simulink subsystem "star_sensor"  (R2022b)
settings: Solver=VariableStepAuto  StartTime=0.0  StopTime=10.0  RelTol=1e-3
undefined symbols (not defined in the file or in its folder): catalogue, sat, sensors
libraries: simulink_extras x1
settings Model: Creator=brent  LastModifiedBy=brent

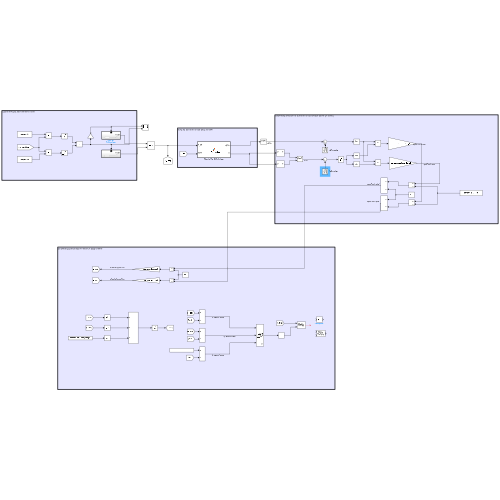
[thumbnail: Simulink's stored preview of the top-level diagram]
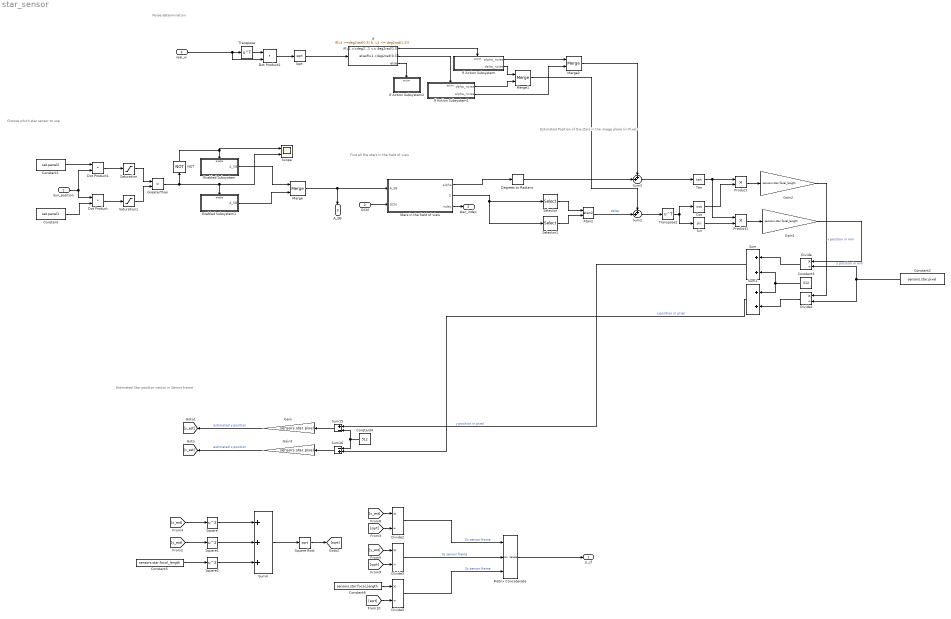
== system star_sensor ==
  note: Noise determination
  note: Estimated Star position vector in Sensor frame
  note: Estimated Position of the stars in the image plane (in Pixel)
  note: Find all the stars in the field of view
  note: Choose which star sensor to use
  Sun_position : Inport
  DCM : Inport  Port=2
  real_w : Inport  Port=3
  Atan2 : Trigonometry  Operator=atan2
  Constant : Constant  Value=sat.panel1
  Constant1 : Constant  Value=sat.panel2
  Constant2 : Constant  Value=sensors.star.pixel
  Constant3 : Constant  Value=512
  Constant4 : Constant  Value=512
  Constant5 : Constant  Value=sensors.star.focal_length
  Constant6 : Constant  Value=sensors.star.focal_length
  Cos : Trigonometry  Operator=cos
  Degrees to Radians : simulink_extras/Transformations/Degrees to Radians
  Divide{,1..3,5} (5 alike) : Product  Inputs=*/
  Dot Product : DotProduct  OutDataTypeStr=Inherit: Inherit via internal rule
  Dot Product1 : DotProduct  OutDataTypeStr=Inherit: Inherit via internal rule
  Dot Product2 : DotProduct  OutDataTypeStr=Inherit: Inherit via internal rule
  Enabled Subsystem : Subsystem  TreatAsAtomicUnit=on
  Enabled Subsystem1 : Subsystem  TreatAsAtomicUnit=on
  Gain : Gain  Gain=sensors.star.pixel
  Gain1 : Gain  Gain=sensors.star.focal_length
  Gain2 : Gain  Gain=sensors.star.focal_length
  Gain3 : Gain  Gain=sensors.star.pixel
  GreaterThan : RelationalOperator  Operator=>  OutDataTypeStr=boolean  RndMeth=Simplest  InputSameDT=off
  If : If  IfExpression="u1 >=deg2rad(0.3) &  u1 <= deg2rad(1.5)"  ElseIfExpressions=u1 <deg2rad(0.3)
  If Action Subsystem : Subsystem  TreatAsAtomicUnit=on
  If Action Subsystem1 : Subsystem  TreatAsAtomicUnit=on
  If Action Subsystem2 : Subsystem  TreatAsAtomicUnit=on
  Matrix Concatenate : Concatenate  NumInputs=3  Mode=Multidimensional array  ConcatenateDimension=2
  Merge : Merge
  Merge1 : Merge
  Merge2 : Merge
  NOT : Logic  Operator=NOT  IconShape=distinctive  AllPortsSameDT=off  OutDataTypeStr=boolean
  Product : Product
  Product1 : Product
  Saturation : Saturate  UpperLimit=1  LowerLimit=0
  Saturation1 : Saturate  UpperLimit=1  LowerLimit=0
  Scope : Scope  NumInputPorts=2
  Selector : Selector  NumberOfDimensions=2  InputPortWidth=3  IndexOptions=Index vector (dialog),Index vector (dialog)  Indices=2,[1:10]  OutputSizes=1,1
  Selector1 : Selector  NumberOfDimensions=2  InputPortWidth=3  IndexOptions=Index vector (dialog),Index vector (dialog)  Indices=1,[1:10]  OutputSizes=1,1
  Sin : Trigonometry
  Sqrt : Sqrt
  Square : Math  Operator=square
  Square Root : Sqrt
  Square1 : Math  Operator=square
  Square2 : Math  Operator=square
  Stars in the field of view : MATLAB Function  TreatAsAtomicUnit=on
  Sum : Sum
  Sum1 : Sum
  Sum15 : Sum  Inputs=+-
  Sum16 : Sum  Inputs=-+
  Sum2 : Sum  Inputs=++|
  Sum3 : Sum  Inputs=++|
  Sum4 : Sum  Inputs=+++
  Tan : Trigonometry  Operator=tan
  Transpose : Math  Operator=transpose
  Transpose2 : Math  Operator=transpose
  si_sf : Outport
  star_index : Outport  Port=2
  A_SB : Outport  Port=3
  wires:
  DCM/1 -> Stars in the field of view/2(DCM)
  Sun_position/1 -> Dot Product/1, Dot Product1/2
  Constant/1 -> Dot Product/2
  Dot Product/1 -> Saturation1/1
  Dot Product1/1 -> Saturation/1
  Constant1/1 -> Dot Product1/1
  Saturation/1 -> GreaterThan/1
  Saturation1/1 -> GreaterThan/2
  GreaterThan/1 -> NOT/1, Enabled Subsystem1/Enable, Scope/2
  NOT/1 -> Enabled Subsystem/Enable, Scope/1
  Enabled Subsystem/1(A_SB) -> Merge/1
  Enabled Subsystem1/1(A_SB) -> Merge/2
  Merge/1 -> Stars in the field of view/1(A_SB), A_SB/1
  Stars in the field of view/1(alpha) -> Degrees to Radians/1
  Tan/1 -> Product/1, Product1/1
  Cos/1 -> Product/2
  Sin/1 -> Product1/2
  Product1/1 -> Gain1/1
  Product/1 -> Gain2/1
  Gain2/1 -> Divide1/1  "x position in mm"
  Gain1/1 -> Divide/1  "y position in mm"
  Constant2/1 -> Divide1/2, Divide/2
  Constant3/1 -> Sum1/1, Sum/2
  Divide1/1 -> Sum1/2
  Divide/1 -> Sum/1
  Sum/1 -> Sum15/1  "y position in pixel"
  Sum1/1 -> Sum16/2  "x position in pixel"
  Stars in the field of view/2(S) -> Selector/1, Selector1/1
  Constant4/1 -> Sum16/1, Sum15/2
  Sum15/1 -> Gain/1
  Sum16/1 -> Gain3/1
  Gain/1 -> [y_est]  "estimated y position"
  Gain3/1 -> [x_est]  "estimated x position"
  [x_est] -> Square/1
  Square/1 -> Sum4/1
  [y_est] -> Square1/1
  Square1/1 -> Sum4/2
  Constant5/1 -> Square2/1
  Square2/1 -> Sum4/3
  Sum4/1 -> Square Root/1
  Square Root/1 -> [sqrt]
  [x_est] -> Divide2/1
  [sqrt] -> Divide2/2
  [sqrt] -> Divide3/2
  [sqrt] -> Divide5/2
  Constant6/1 -> Divide5/1
  [y_est] -> Divide3/1
  Divide2/1 -> Matrix Concatenate/1  "Sx sensor frame"
  Divide3/1 -> Matrix Concatenate/2  "Sy sensor frame"
  Divide5/1 -> Matrix Concatenate/3  "Sz sensor frame"
  Selector/1 -> Atan2/1
  Selector1/1 -> Atan2/2
  Transpose2/1 -> Cos/1, Sin/1
  Sum2/1 -> Transpose2/1
  Degrees to Radians/1 -> Sum3/2
  Sum3/1 -> Tan/1
  Matrix Concatenate/1 -> si_sf/1
  Stars in the field of view/3(index) -> star_index/1
  real_w/1 -> Transpose/1, Dot Product2/2
  Transpose/1 -> Dot Product2/1
  Dot Product2/1 -> Sqrt/1
  If/1 -> If Action Subsystem/Action
  If Action Subsystem/2(delta_noise) -> Merge1/1
  If Action Subsystem1/1(delta_noise) -> Merge1/2
  If Action Subsystem/1(alpha_noise) -> Merge2/1
  If Action Subsystem1/2(alpha_noise) -> Merge2/2
  Atan2/1 -> Sum2/2  "delta"
  Merge2/1 -> Sum3/1
  Merge1/1 -> Sum2/1
  If/2 -> If Action Subsystem1/Action
  If/3 -> If Action Subsystem2/Action
  Sqrt/1 -> If/1

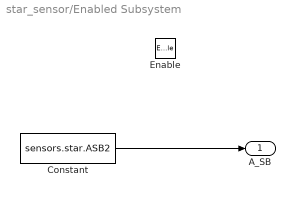
== system star_sensor/Enabled Subsystem ==
  Enable : EnablePort
  Constant : Constant  Value=sensors.star.ASB2
  A_SB : Outport
  wires:
  Constant/1 -> A_SB/1

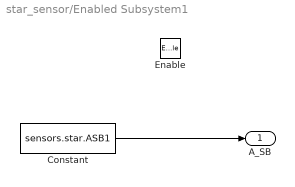
== system star_sensor/Enabled Subsystem1 ==
  Enable : EnablePort
  Constant : Constant  Value=sensors.star.ASB1
  A_SB : Outport
  wires:
  Constant/1 -> A_SB/1

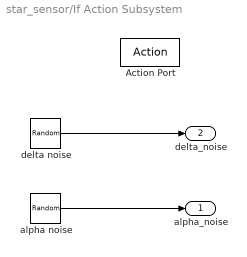
== system star_sensor/If Action Subsystem ==
  Action Port : ActionPort
  "alpha noise " : RandomNumber  Variance=sensors.star.alpha_err*100  Seed=1687
  delta noise : RandomNumber  Variance=sensors.star.delta_err*100  Seed=798
  alpha_noise : Outport
  delta_noise : Outport  Port=2
  wires:
  "alpha noise "/1 -> alpha_noise/1
  delta noise/1 -> delta_noise/1

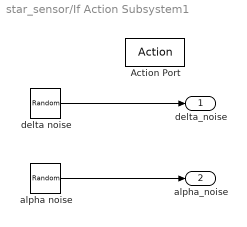
== system star_sensor/If Action Subsystem1 ==
  Action Port : ActionPort
  "alpha noise " : RandomNumber  Variance=sensors.star.alpha_err  Seed=1687
  delta noise : RandomNumber  Variance=sensors.star.delta_err  Seed=798
  delta_noise : Outport
  alpha_noise : Outport  Port=2
  wires:
  delta noise/1 -> delta_noise/1
  "alpha noise "/1 -> alpha_noise/1

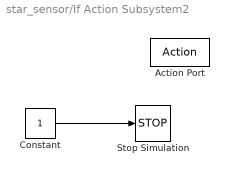
== system star_sensor/If Action Subsystem2 ==
  Action Port : ActionPort
  Constant : Constant
  Stop Simulation : Stop
  wires:
  Constant/1 -> Stop Simulation/1

== matlab function star_sensor/Stars in the field of view ==
  data: alpha output; S output; sensors parameter; catalogue parameter; A_SB input; DCM input; index output
function [alpha,S,index] = findVisibleStars(sensors,catalogue,A_SB,DCM)
%{
    This function takes as an input the star catalogue, the star sensor
    parameters and the current attitude to find the list of visible stars
%}

index = zeros(10,1);

S = sensors.star.S;
alpha = sensors.star.alpha;

i = 1;
j = 1;

while j<=10

    % star's normalized position vector in sensor frame
    S_temp = A_SB*DCM*(catalogue(i,1:3))';
 
    % angle between star's position vector and sensor's pointing axis
    alpha_temp = acos( dot(S_temp,[0;0;1]) );
    alpha_temp = rad2deg(alpha_temp);
    % check if star is in field of view
    if alpha_temp <= sensors.star.fov/2

        S(:,j) = [S_temp;i];
        index (j) = i;
        alpha(j) = alpha_temp;
        j = j + 1;
    end
    i= i+1;
end
